simulink library "DaVinci_LibDynamical"  (R2023a)
settings: Solver=VariableStepAuto  StartTime=0.0  StopTime=10.0  RelTol=1e-3
settings Model: Creator=afons  LastModifiedBy=afons

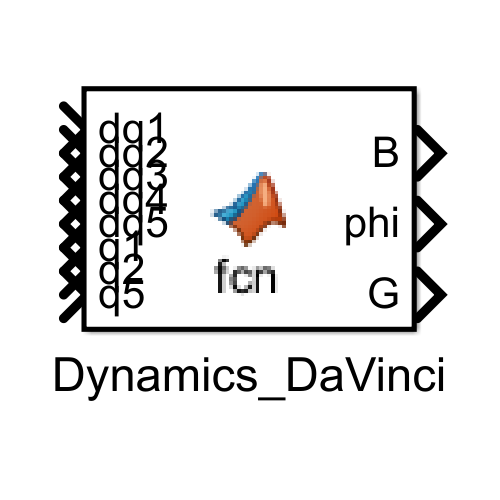
[thumbnail: Simulink's stored preview of the top-level diagram]
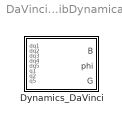
== system DaVinci_LibDynamical ==
  Dynamics_DaVinci : MATLAB Function  TreatAsAtomicUnit=on

== matlab function DaVinci_LibDynamical/Dynamics_DaVinci ==
  data: dq1 input; B output; dq2 input; dq3 input; dq4 input; dq5 input; q1 input; q2 input; q5 input; phi output; G output
function [B,phi,G] = Dynamics_DaVinci(dq1,dq2,dq3,dq4,dq5,q1,q2,q5)
%#codegen

%    This function was generated by the Symbolic Math Toolbox version 9.3.
%    10-Jun-2023 23:51:54

% dq1 = complex(dq1);  % if required to enforce complex operations
% dq2 = complex(dq2);  % if required to enforce complex operations
% dq3 = complex(dq3);  % if required to enforce complex operations
% dq4 = complex(dq4);  % if required to enforce complex operations
% dq5 = complex(dq5);  % if required to enforce complex operations
% q1 = complex(q1);  % if required to enforce complex operations
% q2 = complex(q2);  % if required to enforce complex operations
% q5 = complex(q5);  % if required to enforce complex operations
t2 = cos(q1);
t3 = cos(q2);
t4 = sin(q1);
t5 = sin(q2);
t6 = dq1.^2;
t7 = dq2.^2;
t8 = dq3.^2;
t9 = dq4.^2;
t10 = q2.*2.0;
t11 = q5.^2;
t13 = dq2.*dq5.*q5.*6.0;
t14 = dq3.*dq5.*q5.*6.0;
t15 = dq4.*dq5.*q5.*6.0;
t16 = pi./9.0;
t17 = pi.*(2.0./9.0);
t18 = pi.*(2.0./1.5e+1);
t19 = pi.*(4.0./1.5e+1);
t20 = pi./4.5e+1;
t29 = pi.*(1.1e+1./4.5e+1);
t87 = q5.*1.629681813536099;
t88 = dq2.*dq5.*1.629681813536099;
t89 = dq3.*dq5.*1.629681813536099;
t90 = dq4.*dq5.*1.629681813536099;
t12 = t11.*3.0;
t21 = cos(t16);
t22 = cos(t18);
t23 = cos(t20);
t24 = sin(t16);
t25 = sin(t18);
t26 = sin(t19);
t27 = sin(t20);
t28 = -t20;
t30 = q2+t16;
t31 = q2+t18;
t32 = q2+t19;
t33 = t3.*(5.7e+1./1.6e+2);
t35 = q2+t29;
t41 = t10+t17;
t42 = t10+t19;
t51 = t10+t29;
t91 = -t87;
t92 = -t88;
t93 = -t89;
t94 = -t90;
t34 = q2+t28;
t36 = cos(t30);
t37 = cos(t31);
t38 = sin(t30);
t39 = sin(t31);
t40 = sin(t32);
t44 = cos(t35);
t46 = sin(t35);
t47 = cos(t41);
t48 = sin(t41);
t49 = sin(t42);
t50 = t23.*(3.0./4.0);
t52 = cos(t51);
t53 = sin(t51);
t55 = q5.*t27.*(3.0./4.0);
t60 = q5.*t7.*t23.*(-3.0./4.0);
t61 = q5.*t6.*t23.*(3.0./8.0);
t69 = t6.*t26.*(7.9e+1./4.0e+2);
t80 = t25.*1.283525893800591e+18;
t95 = t23.*1.756088156396867e-2;
t97 = t27.*2.162102266920123e-1;
t98 = t6.*t27.*8.780440781984337e-3;
t99 = t7.*t27.*1.756088156396867e-2;
t103 = t6.*t25.*2.982089252561357e-2;
t109 = t6.*t23.*1.081051133460062e-1;
t110 = t7.*t23.*2.162102266920123e-1;
t43 = cos(t34);
t45 = sin(t34);
t54 = -t50;
t56 = -t55;
t57 = t38.*pi.*(1.1e+1./6.0);
t67 = -t61;
t73 = q5.*t6.*t44.*(9.0./1.0e+1);
t74 = t6.*t11.*t48.*(3.0./2.0);
t76 = q5.*t6.*t52.*(3.0./8.0);
t79 = t38.*6.326974373422939e+16;
t82 = t39.*1.238489897526886e+18;
t83 = t36.*7.789794370910698e+17;
t84 = q5.*t36.*2.702159776422298e+18;
t96 = -t95;
t100 = q5.*t6.*t36.*6.278082636971277e-2;
t108 = -t103;
t118 = t6.*t46.*2.107305787676241e-2;
t119 = q5.*t6.*t48.*8.148409067680494e-1;
t121 = t6.*t44.*2.594522720304148e-1;
t125 = q5.*t6.*t47.*3.768264469190602e-2;
t126 = t6.*t53.*8.780440781984337e-3;
t128 = t6.*t52.*1.081051133460062e-1;
t132 = t6.*t38.*1.46998220848881e-3;
t133 = t6.*t36.*1.809847560174329e-2;
t135 = t6.*t47.*1.186316420158874e-2;
t138 = t6.*t48.*1.153108481011553e-1;
t59 = t43.*(9.0./1.0e+1);
t62 = q5.*t45.*(9.0./5.0);
t63 = dq2.*dq5.*t45.*(9.0./5.0);
t64 = dq3.*dq5.*t45.*(9.0./5.0);
t65 = dq4.*dq5.*t45.*(9.0./5.0);
t68 = q5.*t45.*(9.0./1.0e+1);
t70 = dq2.*dq4.*q5.*t43.*(9.0./5.0);
t71 = dq3.*dq4.*q5.*t43.*(9.0./5.0);
t75 = -t73;
t77 = -t74;
t78 = -t76;
t81 = -t79;
t85 = -t83;
t86 = -t84;
t101 = t43.*2.107305787676241e-2;
t102 = t43.*4.214611575352482e-2;
t104 = t45.*2.594522720304148e-1;
t105 = t45.*5.189045440608296e-1;
t111 = dq2.*dq4.*t45.*4.214611575352482e-2;
t112 = dq3.*dq4.*t45.*4.214611575352482e-2;
t115 = dq2.*dq4.*t43.*5.189045440608296e-1;
t116 = dq3.*dq4.*t43.*5.189045440608296e-1;
t117 = t9.*t45.*2.107305787676241e-2;
t120 = t9.*t43.*2.594522720304148e-1;
t124 = -t118;
t129 = -t126;
t134 = -t133;
t136 = -t135;
t139 = -t138;
t66 = -t59;
t72 = q5.*t9.*t59;
t106 = -t102;
t107 = -t101;
t113 = -t105;
t114 = -t104;
t122 = -t115;
t123 = -t116;
t127 = -t120;
t137 = t79+t84+t85;
t141 = t80+t81+t83+t86;
t130 = t66+3.768264469190602e-2;
t140 = t137.*pi.*6.784696261598179e-19;
t142 = t141.*pi.*6.784696261598179e-19;
t144 = t82+t141;
t147 = t12+t68+t91+t107+t114+2.436887726927406e-1;
t149 = t12+t33+t56+t62+t91+t96+t97+t106+t113+6.461887726927406e-1;
t131 = t54+t130;
t143 = -t142;
t145 = t144.*pi.*6.784696261598179e-19;
t148 = t56+t96+t97+t147;
t146 = -t145;
et1 = q5.*(-8.148409067680494e-1)+t11.*(3.0./2.0)-t22.*5.964178505122713e-2+t33+t36.*2.93996441697762e-3-t37.*6.539669413511747e-2;
et2 = t38.*3.619695120348657e-2-t44.*2.107305787676241e-2-t46.*2.594522720304148e-1;
et3 = t47.*(-1.153108481011553e-1)+t48.*1.186316420158874e-2-t52.*1.756088156396867e-2;
et4 = t53.*(-2.162102266920123e-1)+t56+t68+t96+t97+t107+t114+cos(t19).*(7.9e+1./4.0e+2)+cos(t32).*(5.7e+1./1.6e+2)+cos(t42).*1.8421875e-1-q5.*t38.*1.255616527394255e-1+q5.*t46.*(9.0./1.0e+1)+q5.*t47.*8.148409067680494e-1;
et5 = q5.*t48.*(-3.768264469190602e-2)+q5.*t53.*(3.0./4.0)-t11.*t47.*(3.0./2.0)+pi.^2.*2.054012345679012+5.429425054126636e-1;
mt1 = [et1+et2+et3+et4+et5,t146,t143,t140,t57,t146,t3.*(5.7e+1./8.0e+1)+t12-t23.*3.512176312793735e-2+t27.*4.324204533840247e-1+t62+t91+t106+t113-q5.*t27.*(3.0./2.0)+1.022126272692741,t149,t148,t131,t143,t149];
mt2 = [t12+t62+t91+t106+t113+6.461887726927406e-1,t147,t130,t140,t148,t147,t12+t91+2.436887726927406e-1,3.768264469190602e-2];
mt3 = [t57,t131,t130,3.768264469190602e-2,3.0];
B = reshape([mt1,mt2,mt3],5,5);
if nargout > 1
    et6 = dq1.*dq5.*(-8.148409067680494e-1)-t7.*t22.*pi.*(2.09e+2./2.4e+2)-t8.*t22.*pi.*(2.09e+2./2.4e+2)+t7.*t36.*pi.*4.292659937859009e-2-t7.*t37.*pi.*(1.21e+2./1.44e+2)+t8.*t36.*pi.*4.292659937859009e-2;
    et7 = t7.*t38.*pi.*5.285138874693635e-1+t9.*t36.*pi.*4.292659937859009e-2+t8.*t38.*pi.*5.285138874693635e-1+t9.*t38.*pi.*5.285138874693635e-1+dq1.*dq5.*q5.*3.0+dq1.*dq3.*t5.*(5.7e+1./1.6e+2);
    et8 = dq1.*dq3.*t23.*(-2.162102266920123e-1)+dq1.*dq2.*t25.*5.964178505122713e-2-dq1.*dq4.*t23.*2.162102266920123e-1-dq1.*dq2.*t26.*(7.9e+1./2.0e+2)+dq1.*dq3.*t25.*5.964178505122713e-2-dq1.*dq3.*t26.*(7.9e+1./2.0e+2);
    et9 = dq1.*dq3.*t27.*(-1.756088156396867e-2)-dq1.*dq4.*t27.*1.756088156396867e-2-dq1.*dq5.*t27.*(3.0./4.0)+dq1.*dq2.*t36.*3.619695120348657e-2;
    et10 = dq1.*dq3.*t36.*3.619695120348657e-2-dq1.*dq2.*t38.*2.93996441697762e-3;
    et11 = dq1.*dq4.*t36.*3.619695120348657e-2+dq1.*dq2.*t39.*6.539669413511747e-2-dq1.*dq3.*t38.*2.93996441697762e-3-dq1.*dq2.*t40.*(5.7e+1./8.0e+1);
    et12 = dq1.*dq4.*t38.*(-2.93996441697762e-3)-dq1.*dq3.*t40.*(5.7e+1./1.6e+2)-dq1.*dq5.*t38.*1.255616527394255e-1-dq1.*dq2.*t44.*5.189045440608296e-1;
    et13 = dq1.*dq3.*t44.*(-5.189045440608296e-1)-dq1.*dq4.*t43.*2.594522720304148e-1+dq1.*dq2.*t46.*4.214611575352482e-2-dq1.*dq4.*t44.*2.594522720304148e-1;
    et14 = dq1.*dq2.*t47.*2.372632840317748e-2+dq1.*dq3.*t46.*4.214611575352482e-2+dq1.*dq4.*t45.*2.107305787676241e-2;
    et15 = dq1.*dq2.*t48.*2.306216962023107e-1+dq1.*dq3.*t47.*2.372632840317748e-2+dq1.*dq4.*t46.*2.107305787676241e-2;
    et16 = dq1.*dq5.*t45.*(9.0./1.0e+1)-dq1.*dq2.*t49.*3.684375e-1+dq1.*dq3.*t48.*2.306216962023107e-1+dq1.*dq4.*t47.*2.372632840317748e-2+dq1.*dq5.*t46.*(9.0./1.0e+1);
    et17 = dq1.*dq4.*t48.*2.306216962023107e-1+dq1.*dq5.*t47.*8.148409067680494e-1-dq1.*dq5.*t48.*3.768264469190602e-2;
    et18 = dq1.*dq2.*t52.*(-4.324204533840247e-1)+dq1.*dq2.*t53.*3.512176312793735e-2-dq1.*dq3.*t52.*2.162102266920123e-1+dq1.*dq3.*t53.*1.756088156396867e-2;
    et19 = dq1.*dq4.*t52.*(-2.162102266920123e-1)+dq1.*dq4.*t53.*1.756088156396867e-2+dq1.*dq5.*t53.*(3.0./4.0)-q5.*t7.*t38.*pi.*(1.1e+1./6.0)-q5.*t8.*t38.*pi.*(1.1e+1./6.0)-q5.*t9.*t38.*pi.*(1.1e+1./6.0)-dq1.*dq2.*q5.*t36.*1.255616527394255e-1;
    et20 = dq1.*dq3.*q5.*t36.*(-1.255616527394255e-1)-dq1.*dq4.*q5.*t36.*1.255616527394255e-1+dq1.*dq2.*q5.*t44.*(9.0./5.0)+dq1.*dq3.*q5.*t44.*(9.0./5.0)+dq1.*dq4.*q5.*t44.*(9.0./1.0e+1)-dq1.*dq2.*q5.*t47.*7.536528938381205e-2-dq1.*dq2.*q5.*t48.*1.629681813536099;
    et21 = dq1.*dq3.*q5.*t47.*(-7.536528938381205e-2)-dq1.*dq3.*q5.*t48.*1.629681813536099-dq1.*dq4.*q5.*t47.*7.536528938381205e-2-dq1.*dq4.*q5.*t48.*1.629681813536099-dq1.*dq5.*q5.*t47.*3.0+dq1.*dq3.*q5.*t50+dq1.*dq2.*q5.*t52.*(3.0./2.0)+dq1.*dq4.*q5.*t50+dq1.*dq3.*q5.*t52.*(3.0./4.0);
    et22 = dq1.*dq4.*q5.*t52.*(3.0./4.0)+dq1.*dq4.*q5.*t59+dq1.*dq2.*t12.*t48+dq1.*dq3.*t12.*t48+dq1.*dq4.*t12.*t48-dq2.*dq3.*t22.*pi.*(2.09e+2./1.2e+2)+dq2.*dq3.*t36.*pi.*8.585319875718019e-2+dq2.*dq4.*t36.*pi.*8.585319875718019e-2+dq2.*dq3.*t38.*pi.*1.057027774938727+dq2.*dq5.*t36.*pi.*(1.1e+1./3.0);
    et23 = dq3.*dq4.*t36.*pi.*8.585319875718019e-2+dq2.*dq4.*t38.*pi.*1.057027774938727+dq3.*dq5.*t36.*pi.*(1.1e+1./3.0)+dq3.*dq4.*t38.*pi.*1.057027774938727+dq4.*dq5.*t36.*pi.*(1.1e+1./3.0)-dq2.*dq3.*q5.*t38.*pi.*(1.1e+1./3.0)-dq2.*dq4.*q5.*t38.*pi.*(1.1e+1./3.0)-dq3.*dq4.*q5.*t38.*pi.*(1.1e+1./3.0);
    et24 = t13+t14+t15+t63+t64+t65+t69+t70+t71+t72+t75+t77+t92+t93+t94+t100+t108+t111+t112+t117+t119+t121+t122+t123+t124+t125+t127+t132+t134+t136+t139+t5.*t8.*(5.7e+1./1.6e+2)-t8.*t23.*2.162102266920123e-1-t9.*t23.*2.162102266920123e-1-t8.*t27.*1.756088156396867e-2;
    et25 = t9.*t27.*(-1.756088156396867e-2)-t6.*t39.*3.269834706755874e-2+t6.*t40.*(5.7e+1./1.6e+2)+t6.*t49.*1.8421875e-1+t6.*t52.*2.162102266920123e-1-t6.*t53.*1.756088156396867e-2+dq2.*dq3.*t5.*(5.7e+1./8.0e+1);
    et26 = dq2.*dq3.*t23.*(-4.324204533840247e-1)-dq2.*dq4.*t23.*4.324204533840247e-1-dq3.*dq4.*t23.*4.324204533840247e-1-dq2.*dq3.*t27.*3.512176312793735e-2;
    et27 = dq2.*dq4.*t27.*(-3.512176312793735e-2)-dq2.*dq5.*t27.*(3.0./2.0)-dq3.*dq4.*t27.*3.512176312793735e-2-dq3.*dq5.*t27.*(3.0./2.0)-dq4.*dq5.*t27.*(3.0./2.0)-q5.*t6.*t52.*(3.0./4.0)+q5.*t8.*t50+q5.*t9.*t50+dq2.*dq3.*q5.*t23.*(3.0./2.0)+dq2.*dq4.*q5.*t23.*(3.0./2.0)+dq3.*dq4.*q5.*t23.*(3.0./2.0);
    et28 = t13+t14+t15+t60+t67+t77+t78+t92+t93+t94+t98+t99+t100+t109+t110+t119+t125+t128+t129+t132+t134+t136+t139+t6.*t43.*1.297261360152074e-1+t6.*t44.*1.297261360152074e-1+t7.*t43.*2.594522720304148e-1-t6.*t45.*1.05365289383812e-2;
    et29 = t8.*t43.*2.594522720304148e-1-t6.*t46.*1.05365289383812e-2-t7.*t45.*2.107305787676241e-2-t8.*t45.*2.107305787676241e-2;
    et30 = dq2.*dq3.*t43.*5.189045440608296e-1-dq2.*dq3.*t45.*4.214611575352482e-2-q5.*t6.*t43.*(9.0./2.0e+1)-q5.*t6.*t44.*(9.0./2.0e+1)-q5.*t7.*t43.*(9.0./1.0e+1)-q5.*t8.*t43.*(9.0./1.0e+1)-dq2.*dq3.*q5.*t43.*(9.0./5.0);
    et31 = t6.*4.074204533840247e-1+t7.*8.148409067680494e-1+t8.*8.148409067680494e-1+t9.*8.148409067680494e-1+dq2.*dq3.*1.629681813536099;
    et32 = dq2.*dq4.*1.629681813536099+dq3.*dq4.*1.629681813536099-q5.*t6.*(3.0./2.0)-q5.*t7.*3.0-q5.*t8.*3.0-q5.*t9.*3.0+t6.*t27.*(3.0./8.0)+t7.*t27.*(3.0./4.0)+t6.*t38.*6.278082636971277e-2-t6.*t45.*(9.0./2.0e+1)-t6.*t46.*(9.0./2.0e+1)-t7.*t45.*(9.0./1.0e+1);
    et33 = t6.*t47.*(-4.074204533840247e-1)-t8.*t45.*(9.0./1.0e+1)+t6.*t48.*1.884132234595301e-2-t6.*t53.*(3.0./8.0)-dq2.*dq3.*q5.*6.0-dq2.*dq4.*q5.*6.0-dq3.*dq4.*q5.*6.0-dq2.*dq3.*t45.*(9.0./5.0)+q5.*t6.*t47.*(3.0./2.0);
    phi = [et6+et7+et8+et9+et10+et11+et12+et13+et14+et15+et16+et17+et18+et19+et20+et21+et22+et23;et24+et25+et26+et27;t13+t14+t15+t60+t63+t64+t65+t67+t69+t70+t71+t72+t75+t77+t78+t92+t93+t94+t98+t99+t100+t108+t109+t110+t111+t112+t117+t119+t121+t122+t123+t124+t125+t127+t128+t129+t132+t134+t136+t139-t5.*t6.*(5.7e+1./3.2e+2)-t5.*t7.*(5.7e+1./1.6e+2)+t6.*t40.*(5.7e+1./3.2e+2);et28+et29+et30;et31+et32+et33];
end
if nargout > 2
    et34 = t2.*(-2.052933022289608)+t4.*pi.*3.29725e+1+t2.*t22.*1.397925e+1-t2.*t3.*t21.*6.890889925701308e-1+t2.*t3.*t22.*(9.81e+2./6.4e+1)-t2.*t5.*t21.*8.484089295394564;
    et35 = t2.*t3.*t24.*(-8.484089295394564)+t2.*t5.*t24.*6.890889925701308e-1-t2.*t5.*t25.*(9.81e+2./6.4e+1)+q5.*t2.*t5.*t21.*2.943e+1+q5.*t2.*t3.*t24.*2.943e+1;
    G = [et34+et35;t4.*(t39.*1.40737488355328e+18+t141).*(-1.089128787157279e-17);t4.*t141.*(-1.089128787157279e-17);t4.*t137.*1.089128787157279e-17;t4.*t38.*2.943e+1];
end
end
